simulink model "generic"  (R2022b)
settings: Solver=ode45  StartTime=0.0  StopTime=inf  RelTol=1e-3  EnableMultiTasking=on
values from neighbouring files (symbols this model uses):
  A = cell2mat(A_cell)    [MPCController1.m]    (also in MPC_Fmincon.m)
  B = cell2mat(B_cell)    [MPCController1.m]    (also in MPC_Fmincon.m)
  brake_select = ones(length(speed), length(steering_angle))    [TwoDLook_uptable.m]
  curvature = 0.000:0.001:1    [TwoDLook_uptable.m]
  m = 1600    [MPCController1.m]    (also in MPCController2.m; MPC_Fmincon.m)
  speed = 0:0.1:100    [TwoDLook_uptable.m]
undefined symbols (not defined in the file or in its folder): Amplifier, DiscIntNeverNeededParam, K_d_yawrate, K_dsteering, k_speed, k_stanley, kd, ki, kp, path_curvature
libraries: CarMaker4SL x97, simulink x6, cstblocks x6, simulink_extras x4, autolibshared x1, mpcadaslib x1
(part 2 of 6)

== system generic/CarMaker/VehicleControl/CreateBus VhclCtrl1/MPC_steering_controllers ==
  Lateral_dev : Inport
  Dev_angle : Inport  Port=2
  Amplifyer : Gain  Gain=Amplifier
  Amplifyer1 : Gain  Gain=2
  Amplifyer2 : Gain  Gain=-3
  Bus Selector1 : BusSelector  OutputSignals=Path.tx,Path.ty,Path,Path.DevAng,Path.CurveXY
  Constant1 : Constant  Value=3
  Constant2 : Constant  Value=0
  Demux : Demux  Outputs=5
  Discrete-Time Integrator : DiscreteIntegrator  SampleTime=-1  ICPrevOutput=DiscIntNeverNeededParam  ICPrevScaledInput=DiscIntNeverNeededParam
  MATLAB System : MATLABSystem  Commented=on  System=MPCController  Nx=5  Nu=1  Ny=2  Np=20  Nc=10  T=0.01  lf=1.488  lr=1.487  Ccf=66900  Ccr=62700  m=1600  g=9.81  I=2986.624  x_dot=15  Q=diag( [ 2000, 0, 0, 10000, 0 ] )  R=5 * 10 ^ 5  Row=1000  umin=-0.6  umax=0.6  delta_umin=-0.06  delta_umax=0.06  ycmax=[ 0.2; 1000 ]  ycmin=[ -0.2; -1000 ]  SimulateUsing=Code generation
      mask Type: MPCController
      mask Display:
      | disp('MPCController');
      | port_label('input',1,'y_dot');
      | port_label('input',2,'phi');
      | port_label('input',3,'phi_dot');
      | port_label('input',4,'Y');
      | port_label('input',5,'X');
      | port_label('output',1,'delta_f');
      | port_label('output',2,'state_k1');
  Multiport Switch : MultiPortSwitch  SaturateOnIntegerOverflow=off  InputSameDT=off
  Mux1 : Mux  Inputs=5
  Mux3 : Mux  Inputs=1
  Product : Product
  Radians to Degrees : simulink_extras/Transformations/Radians to Degrees
  Radians to Degrees1 : simulink_extras/Transformations/Radians to Degrees
  Read CM Dict : CarMaker4SL/Read CM Dict  xname=Sensor.Road.VehSensor_0.Path.DevAng  xsync=off  xstime=Continuous
  Read CM Dict1 : CarMaker4SL/Read CM Dict  xname=Car.Road.Path.DevDist  xsync=off  xstime=Continuous
  Read CM Dict8 : CarMaker4SL/Read CM Dict  xname=Vhcl.v  xsync=off  xstime=Continuous
  Road Sensor1 : CarMaker4SL/Sensors/Road Sensor  xname=0  xstime=Continuous
      settings: SourceProductName=CarMaker4SL
  S-Function1 : S-Function  Commented=on  FunctionName=MPC_Fmincon  SFunctionDeploymentMode=off  EnableBusSupport=off
  State_space_system_variables : Subsystem
  Subsystem : Subsystem  Commented=on
  Terminator : Terminator
  Terminator1 : Terminator  Commented=on
  Terminator2 : Terminator
  Terminator3 : Terminator
  Tradition_MPC : Subsystem
  steering : Outport
  wires:
  Constant2/1 -> Road Sensor1/1
  Demux/1 -> MATLAB System/4
  Bus Selector1/5 -> Product/2  "<CurveXY>"
  Bus Selector1/3 -> Terminator1/1  "<Path>"
  Road Sensor1/1 -> Terminator/1
  Road Sensor1/2 -> Bus Selector1/1
  Mux3/1 -> S-Function1/1, Demux/1
  Read CM Dict8/1 -> Product/1
  Bus Selector1/1 -> Mux1/5  "<tx>"
  Bus Selector1/2 -> State_space_system_variables/2(<ty>), Mux1/4  "<ty>"
  Product/1 -> Discrete-Time Integrator/1, Radians to Degrees1/1
  Discrete-Time Integrator/1 -> Radians to Degrees/1
  Radians to Degrees/1 -> State_space_system_variables/1(Yaw_ref_deg), Mux1/2
  Constant1/1 -> Multiport Switch/1
  Radians to Degrees1/1 -> Mux1/3
  State_space_system_variables/1(x) -> Mux3/1
  Demux/5 -> MATLAB System/3
  Demux/3 -> MATLAB System/1
  State_space_system_variables/2(Lateral_velocity) -> Mux1/1
  Read CM Dict/1 -> Amplifyer/1
  Mux1/1 -> Terminator2/1  "u"
  Read CM Dict1/1 -> ?
  Amplifyer/1 -> ?  "Dev_angle"
  Demux/2 -> MATLAB System/5
  Demux/4 -> MATLAB System/2
  Amplifyer1/1 -> Tradition_MPC/1(Lateral_deviation)  "Dev_angle"
  Amplifyer2/1 -> Tradition_MPC/2(Dev_angle)  "Dev_angle"
  MATLAB System/1 -> Multiport Switch/3
  Multiport Switch/1 -> steering/1
  MATLAB System/2 -> Terminator3/1
  S-Function1/1 -> Multiport Switch/2
  Tradition_MPC/1(steering_cmd) -> Multiport Switch/4
  Lateral_dev/1 -> Amplifyer1/1
  Dev_angle/1 -> Amplifyer2/1

== system generic/CarMaker/VehicleControl/CreateBus VhclCtrl1/PID steering controller ==
  Lateral_error : Inport
  Add : Sum  Inputs=+++
  Dervative : Subsystem
  Discrete-Time Integrator : DiscreteIntegrator  SampleTime=-1  ICPrevOutput=DiscIntNeverNeededParam  ICPrevScaledInput=DiscIntNeverNeededParam
  Gain : Gain  Gain=1.1
  Gain1 : Gain  Gain=0.9
  steering_cmd : Outport
  wires:
  Lateral_error/1 -> Gain1/1, Gain/1, Dervative/1(Error)
  Discrete-Time Integrator/1 -> Add/1
  Gain1/1 -> Discrete-Time Integrator/1
  Gain/1 -> Add/2
  Add/1 -> steering_cmd/1
  Dervative/1(Dervative term) -> Add/3

== system generic/CarMaker/VehicleControl/CreateBus VhclCtrl1/Smoothing ==
  Signal_In : Inport
  Add : Sum  Inputs=++++
  Delay : Delay  InitialCondition=0.1
  Delay1 : Delay  DelayLength=4  InitialCondition=0.1
  Delay2 : Delay  DelayLength=5  InitialCondition=0.1
  Gain : Gain  Gain=0.35
  Gain1 : Gain  Gain=0.25
  Gain2 : Gain  Gain=0.25
  Gain3 : Gain  Gain=0.15
  Signal_Out : Outport  VectorParamsAs1DForOutWhenUnconnected=off
  wires:
  Gain1/1 -> Add/2
  Signal_In/1 -> Gain/1
  Delay/1 -> Gain1/1
  Gain/1 -> Add/1
  Delay1/1 -> Gain2/1
  Add/1 -> Delay2/1, Delay1/1, Delay/1, Signal_Out/1
  Gain2/1 -> Add/3
  Delay2/1 -> Gain3/1
  Gain3/1 -> Add/4

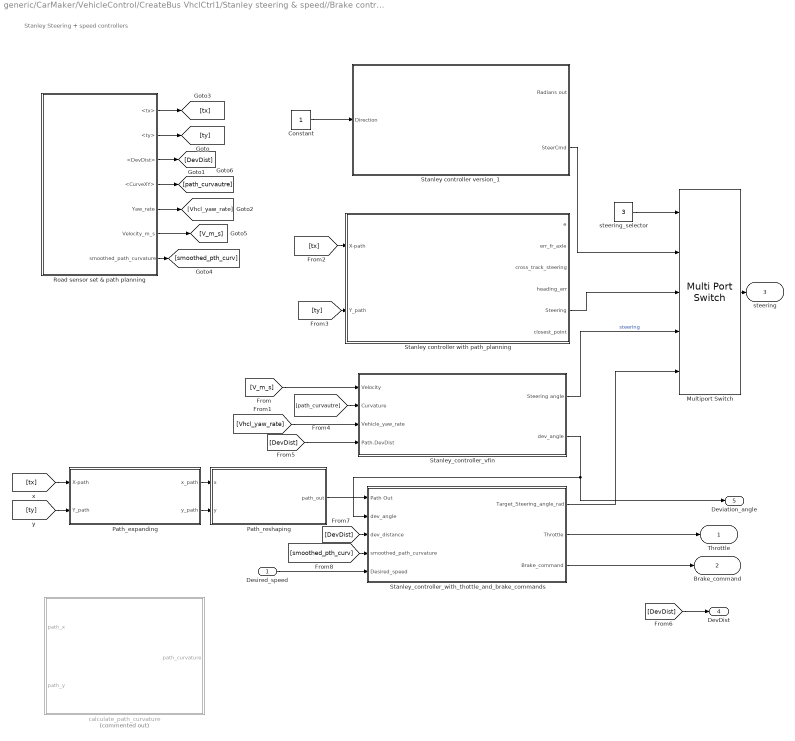
== system generic/CarMaker/VehicleControl/CreateBus VhclCtrl1/Stanley steering & speed//Brake controller ==
  note: Stanley Steering + speed controllers
  Desired_speed : Inport
  " Path_expanding" : Subsystem
  Constant : Constant
  Multiport Switch : MultiPortSwitch  Inputs=4  SaturateOnIntegerOverflow=off  InputSameDT=off
  Path_reshaping : MATLAB Function  TreatAsAtomicUnit=on
  Road sensor set & path planning : Subsystem  Variant=on  VariantControlMode=label  VariantControl=Choice  LabelModeActiveChoice=Choice
  Stanley controller version_1 : Subsystem  Variant=on  VariantControlMode=label  VariantControl=Choice  LabelModeActiveChoice=Choice
  Stanley controller with path_planning : Subsystem  Variant=on  VariantControlMode=label  VariantControl=Choice  LabelModeActiveChoice=Choice
  Stanley_controller_vfin : Subsystem  Variant=on  VariantControlMode=label  VariantControl=Choice  LabelModeActiveChoice=Choice
  Stanley_controller_with_thottle_and_brake_commands : Subsystem
  calculate_path_curvature : Subsystem  Commented=on  Variant=on  VariantControlMode=label  VariantControl=Choice  LabelModeActiveChoice=Choice
  steering_selector : Constant  Value=3
  Throttle : Outport
  Brake_command : Outport  Port=2
  steering : Outport  Port=3
  DevDist : Outport  Port=4
  Deviation_angle : Outport  Port=5
  wires:
  [tx] -> " Path_expanding"/1(X-path)
  [ty] -> " Path_expanding"/2(Y_path)
  [tx] -> Stanley controller with path_planning/1(X-path)
  [ty] -> Stanley controller with path_planning/2(Y_path)
  Road sensor set & path planning/1(<tx>) -> [tx]
  Road sensor set & path planning/2(<ty>) -> [ty]
  Road sensor set & path planning/3(<DevDist>) -> [DevDist]
  Road sensor set & path planning/4(<CurveXY>) -> [path_curvautre]
  Road sensor set & path planning/5(Yaw_rate) -> [Vhcl_yaw_rate]
  [path_curvautre] -> Stanley_controller_vfin/2(Curvature)
  Stanley_controller_vfin/1(Steering angle) -> Multiport Switch/4  "steering"
  Constant/1 -> Stanley controller version_1/1(Direction)
  steering_selector/1 -> Multiport Switch/1
  Stanley controller version_1/2(SteerCmd) -> Multiport Switch/2
  Stanley controller with path_planning/5(Steering) -> Multiport Switch/3
  Path_reshaping/1(path_out) -> Stanley_controller_with_thottle_and_brake_commands/1(Path Out)
  Stanley_controller_vfin/2(dev_angle) -> Deviation_angle/1, Stanley_controller_with_thottle_and_brake_commands/2(dev_angle)
  " Path_expanding"/1(x_path) -> Path_reshaping/1(x)
  " Path_expanding"/2(y_path) -> Path_reshaping/2(y)
  Stanley_controller_with_thottle_and_brake_commands/2(Throttle) -> Throttle/1
  Stanley_controller_with_thottle_and_brake_commands/3(Brake_command) -> Brake_command/1
  Stanley_controller_with_thottle_and_brake_commands/1(Target_Steering_angle_rad) -> Multiport Switch/5
  [V_m_s] -> Stanley_controller_vfin/1(Velocity)
  [Vhcl_yaw_rate] -> Stanley_controller_vfin/3(Vehicle_yaw_rate)
  [DevDist] -> Stanley_controller_vfin/4(Path.DevDist)
  Road sensor set & path planning/6(Velocity_m_s) -> [V_m_s]
  [DevDist] -> DevDist/1
  Multiport Switch/1 -> steering/1
  [DevDist] -> Stanley_controller_with_thottle_and_brake_commands/3(dev_distance)
  Road sensor set & path planning/7(smoothed_path_curvature) -> [smoothed_pth_curv]
  [smoothed_pth_curv] -> Stanley_controller_with_thottle_and_brake_commands/4(smoothed_path_curvature)
  Desired_speed/1 -> Stanley_controller_with_thottle_and_brake_commands/5(Desired_speed)

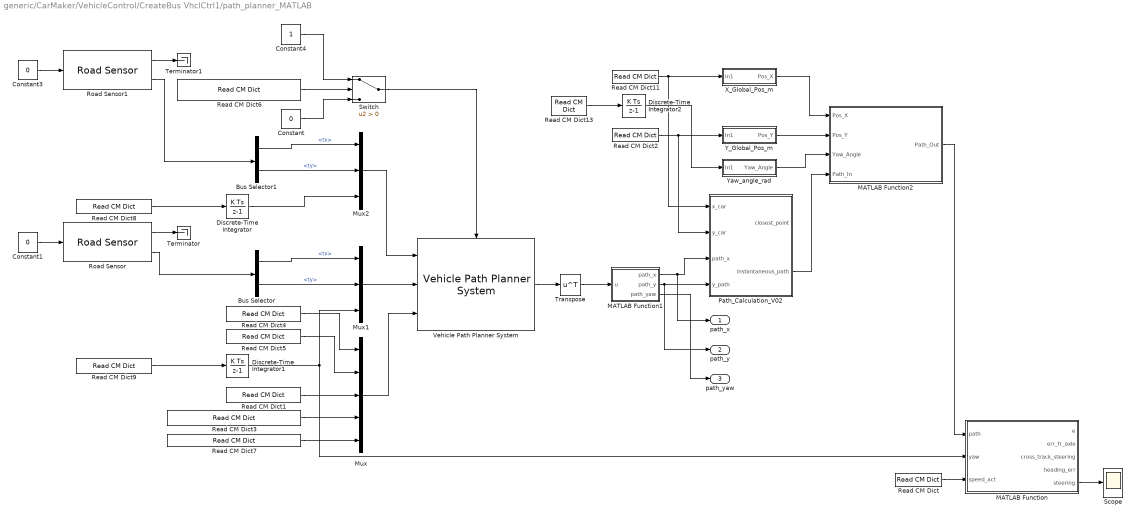
== system generic/CarMaker/VehicleControl/CreateBus VhclCtrl1/path_planner_MATLAB ==
  Bus Selector : BusSelector  OutputSignals=Path.tx,Path.ty
  Bus Selector1 : BusSelector  OutputSignals=Path.tx,Path.ty
  Constant : Constant  Value=0
  Constant1 : Constant  Value=0
  Constant3 : Constant  Value=0
  Constant4 : Constant
  Discrete-Time Integrator : DiscreteIntegrator  SampleTime=-1  ICPrevOutput=DiscIntNeverNeededParam  ICPrevScaledInput=DiscIntNeverNeededParam
  Discrete-Time Integrator1 : DiscreteIntegrator  SampleTime=-1  ICPrevOutput=DiscIntNeverNeededParam  ICPrevScaledInput=DiscIntNeverNeededParam
  Discrete-Time Integrator2 : DiscreteIntegrator  SampleTime=-1  ICPrevOutput=DiscIntNeverNeededParam  ICPrevScaledInput=DiscIntNeverNeededParam
  MATLAB Function : MATLAB Function  TreatAsAtomicUnit=on
  MATLAB Function1 : MATLAB Function  TreatAsAtomicUnit=on
  MATLAB Function2 : MATLAB Function  TreatAsAtomicUnit=on
  Mux : Mux  Inputs=5
  Mux1 : Mux  Inputs=3
  Mux2 : Mux  Inputs=3
  Path_Calculation_V02 : MATLAB Function  TreatAsAtomicUnit=on
  Read CM Dict : CarMaker4SL/Read CM Dict  xname=Vhcl.v  xsync=off  xstime=Continuous
  Read CM Dict1 : CarMaker4SL/Read CM Dict  xname=Traffic.T00.rz  xsync=off  xstime=Continuous
  Read CM Dict11 : CarMaker4SL/Read CM Dict  xname=Car.Gen.tx  xsync=off  xstime=Continuous
  Read CM Dict13 : CarMaker4SL/Read CM Dict  xname=Car.YawRate  xsync=off  xstime=Continuous
  Read CM Dict2 : CarMaker4SL/Read CM Dict  xname=Car.Gen.ty  xsync=off  xstime=Continuous
  Read CM Dict3 : CarMaker4SL/Read CM Dict  xname=Sensor.Radar.VehSensor_6.Obj0.Length  xsync=off  xstime=Continuous
  Read CM Dict4 : CarMaker4SL/Read CM Dict  xname=Traffic.T00.tx  xsync=off  xstime=Continuous
  Read CM Dict5 : CarMaker4SL/Read CM Dict  xname=Traffic.T00.ty  xsync=off  xstime=Continuous
  Read CM Dict6 : CarMaker4SL/Read CM Dict  xname=Sensor.Radar.VehSensor_6.Obj0.ProbObst  xsync=off  xstime=Continuous
  Read CM Dict7 : CarMaker4SL/Read CM Dict  xname=Sensor.Radar.VehSensor_6.Obj0.Width  xsync=off  xstime=Continuous
  Read CM Dict8 : CarMaker4SL/Read CM Dict  xname=Car.YawRate  xsync=off  xstime=Continuous
  Read CM Dict9 : CarMaker4SL/Read CM Dict  xname=Car.YawRate  xsync=off  xstime=Continuous
  Road Sensor : CarMaker4SL/Sensors/Road Sensor  xname=0  xstime=Continuous
      settings: SourceProductName=CarMaker4SL
  Road Sensor1 : CarMaker4SL/Sensors/Road Sensor  xname=0  xstime=Continuous
      settings: SourceProductName=CarMaker4SL
  Scope : Scope
  Switch : Switch  Criteria=u2 > Threshold  SaturateOnIntegerOverflow=off  InputSameDT=off
  Terminator : Terminator
  Terminator1 : Terminator
  Transpose : Math  Operator=transpose
  Vehicle Path Planner System : mpcadaslib/Vehicle Path Planner System  egoLength=4.7  egoWidth=1.8  wheelbase=2.8  dist2Center=1.4  numObs=1  obsMat=zeros(1,5)  obs_ext=on  minDist=1  Ts=1  pPlanning=20  v_range=[-20,30]  v_ext=off  steer_range=[-pi/4,pi/4]  steer_ext=off  suboptimal=off  maxiter=200  output_exitflag=off
      settings: LibrarySourceBlock=mpclib/Automated Driving/Vehicle Path Planner System
  X_Global_Pos_m : Subsystem
  Y_Global_Pos_m : Subsystem
  Yaw_angle_rad : Subsystem
  path_x : Outport
  path_y : Outport  Port=2
  path_yaw : Outport  Port=3
  wires:
  Constant3/1 -> Road Sensor1/1
  Mux1/1 -> Vehicle Path Planner System/2
  Road Sensor/1 -> Terminator/1
  Road Sensor1/1 -> Terminator1/1
  Constant1/1 -> Road Sensor/1
  Bus Selector1/2 -> Mux2/2  "<ty>"
  Read CM Dict9/1 -> Discrete-Time Integrator1/1
  Road Sensor/2 -> Bus Selector/1
  Road Sensor1/2 -> Bus Selector1/1
  Read CM Dict8/1 -> Discrete-Time Integrator/1
  MATLAB Function2/1(Path_Out) -> MATLAB Function/1(path)
  Constant4/1 -> Switch/1
  Read CM Dict6/1 -> Switch/2
  Constant/1 -> Switch/3
  MATLAB Function1/1(path_x) -> Path_Calculation_V02/3(path_x), path_x/1
  Bus Selector1/1 -> Mux2/1  "<tx>"
  Discrete-Time Integrator/1 -> Mux2/3
  Bus Selector/1 -> Mux1/1  "<tx>"
  Bus Selector/2 -> Mux1/2  "<ty>"
  X_Global_Pos_m/1(Pos_X) -> MATLAB Function2/1(Pos_X)
  Read CM Dict4/1 -> Mux/1
  Read CM Dict5/1 -> Mux/2
  Read CM Dict11/1 -> Path_Calculation_V02/1(x_car), X_Global_Pos_m/1(In1)
  Discrete-Time Integrator1/1 -> MATLAB Function/2(yaw), Mux1/3
  Read CM Dict1/1 -> Mux/3
  Read CM Dict3/1 -> Mux/4
  Y_Global_Pos_m/1(Pos_Y) -> MATLAB Function2/2(Pos_Y)
  Read CM Dict7/1 -> Mux/5
  Transpose/1 -> MATLAB Function1/1(u)
  Switch/1 -> Vehicle Path Planner System/Enable
  Mux2/1 -> Vehicle Path Planner System/1
  Mux/1 -> Vehicle Path Planner System/3
  Vehicle Path Planner System/1 -> Transpose/1
  Read CM Dict13/1 -> Discrete-Time Integrator2/1
  Discrete-Time Integrator2/1 -> Yaw_angle_rad/1(In1)
  Read CM Dict2/1 -> Path_Calculation_V02/2(y_car), Y_Global_Pos_m/1(In1)
  MATLAB Function/5(steering) -> Scope/1
  MATLAB Function1/2(path_y) -> path_y/1, Path_Calculation_V02/4(y_path)
  MATLAB Function1/3(path_yaw) -> path_yaw/1
  Yaw_angle_rad/1(Yaw_Angle) -> MATLAB Function2/3(Yaw_Angle)
  Path_Calculation_V02/2(instantaneous_path) -> MATLAB Function2/4(Path_In)
  Read CM Dict/1 -> MATLAB Function/3(speed_act)

== system generic/CarMaker/IPG Vehicle/CarAndTrailer/CarAndTrailerUpd/CreateBus Brake.IF.In ==
  In : Inport
  BusCreator : BusCreator  Inputs=9
  Demux : Demux  Outputs=9
      settings: DisplayOption=none
  Out : Outport  VectorParamsAs1DForOutWhenUnconnected=off
  wires:
  Demux/9 -> BusCreator/9  "Brake IF Trq_Reg RR"
  Demux/8 -> BusCreator/8  "Brake IF Trq_Reg RL"
  Demux/7 -> BusCreator/7  "Brake IF Trq_Reg FR"
  Demux/6 -> BusCreator/6  "Brake IF Trq_Reg FL"
  Demux/5 -> BusCreator/5  "Brake IF Trq_Reg_max RR"
  Demux/4 -> BusCreator/4  "Brake IF Trq_Reg_max RL"
  Demux/3 -> BusCreator/3  "Brake IF Trq_Reg_max FR"
  Demux/2 -> BusCreator/2  "Brake IF Trq_Reg_max FL"
  Demux/1 -> BusCreator/1  "Brake IF T_env"
  BusCreator/1 -> Out/1
  In/1 -> Demux/1

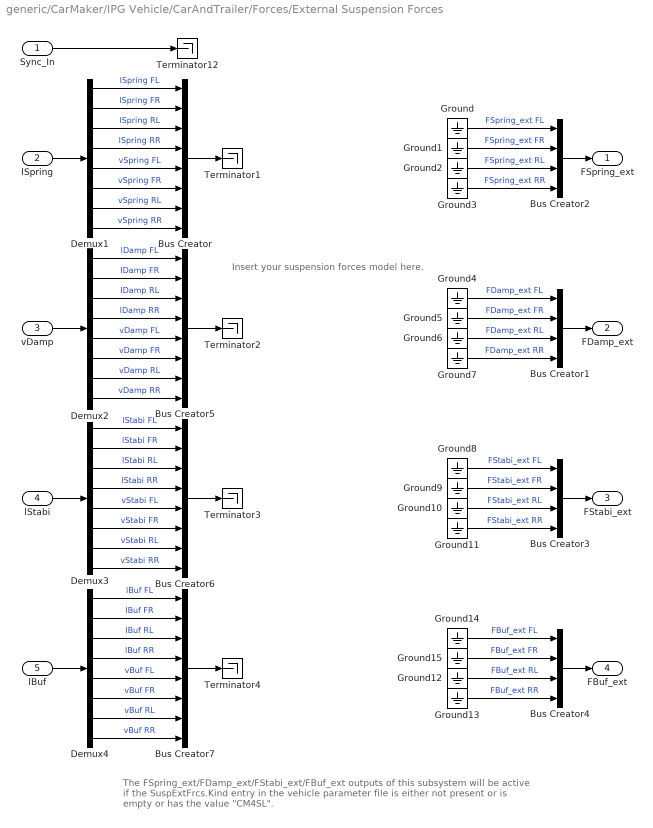
== system generic/CarMaker/IPG Vehicle/CarAndTrailer/Forces/External Suspension Forces ==
  note: The FSpring_ext/FDamp_ext/FStabi_ext/FBuf_ext outputs of this subsystem will be
      | active if the SuspExtFrcs.Kind entry in the vehicle parameter file
      | is either not present or is empty or has the value "CM4SL".
  note: Insert your suspension forces model here.
  Sync_In : Inport
  lSpring : Inport  Port=2
  vDamp : Inport  Port=3
  lStabi : Inport  Port=4
  lBuf : Inport  Port=5
  Bus Creator{,5..7} (4 alike) : BusCreator  Inputs=8
  Bus Creator{1..4} (4 alike) : BusCreator  Inputs=4
  Demux{1..4} (4 alike) : Demux  Outputs=8
      settings: DisplayOption=none
  Ground{,1..15} (16 alike) : Ground
  Terminator{1..4,12} (5 alike) : Terminator
  FSpring_ext : Outport  VectorParamsAs1DForOutWhenUnconnected=off
  FDamp_ext : Outport  Port=2  VectorParamsAs1DForOutWhenUnconnected=off
  FStabi_ext : Outport  Port=3  VectorParamsAs1DForOutWhenUnconnected=off
  FBuf_ext : Outport  Port=4  VectorParamsAs1DForOutWhenUnconnected=off
  wires:
  Bus Creator7/1 -> Terminator4/1
  Bus Creator6/1 -> Terminator3/1
  Bus Creator5/1 -> Terminator2/1
  Bus Creator/1 -> Terminator1/1
  Demux4/8 -> Bus Creator7/8  "vBuf RR"
  Demux4/7 -> Bus Creator7/7  "vBuf RL"
  Demux4/6 -> Bus Creator7/6  "vBuf FR"
  Demux4/5 -> Bus Creator7/5  "vBuf FL"
  Demux3/8 -> Bus Creator6/8  "vStabi RR"
  Demux3/7 -> Bus Creator6/7  "vStabi RL"
  Demux3/6 -> Bus Creator6/6  "vStabi FR"
  Demux3/5 -> Bus Creator6/5  "vStabi FL"
  Demux2/8 -> Bus Creator5/8  "vDamp RR"
  Demux2/7 -> Bus Creator5/7  "vDamp RL"
  Demux2/6 -> Bus Creator5/6  "vDamp FR"
  Demux2/5 -> Bus Creator5/5  "vDamp FL"
  Demux1/8 -> Bus Creator/8  "vSpring RR"
  Demux1/7 -> Bus Creator/7  "vSpring RL"
  Demux1/6 -> Bus Creator/6  "vSpring FR"
  Demux1/5 -> Bus Creator/5  "vSpring FL"
  Demux2/4 -> Bus Creator5/4  "lDamp RR"
  Demux2/3 -> Bus Creator5/3  "lDamp RL"
  Demux2/2 -> Bus Creator5/2  "lDamp FR"
  Demux2/1 -> Bus Creator5/1  "lDamp FL"
  Demux1/4 -> Bus Creator/4  "lSpring RR"
  Demux1/3 -> Bus Creator/3  "lSpring RL"
  Demux1/2 -> Bus Creator/2  "lSpring FR"
  Demux1/1 -> Bus Creator/1  "lSpring FL"
  Demux3/4 -> Bus Creator6/4  "lStabi RR"
  Demux3/3 -> Bus Creator6/3  "lStabi RL"
  Demux3/2 -> Bus Creator6/2  "lStabi FR"
  Demux3/1 -> Bus Creator6/1  "lStabi FL"
  lStabi/1 -> Demux3/1
  vDamp/1 -> Demux2/1
  lSpring/1 -> Demux1/1
  Demux4/4 -> Bus Creator7/4  "lBuf RR"
  Demux4/3 -> Bus Creator7/3  "lBuf RL"
  Demux4/2 -> Bus Creator7/2  "lBuf FR"
  Demux4/1 -> Bus Creator7/1  "lBuf FL"
  lBuf/1 -> Demux4/1
  Ground14/1 -> Bus Creator4/1  "FBuf_ext FL"
  Ground15/1 -> Bus Creator4/2  "FBuf_ext FR"
  Ground12/1 -> Bus Creator4/3  "FBuf_ext RL"
  Ground13/1 -> Bus Creator4/4  "FBuf_ext RR"
  Bus Creator4/1 -> FBuf_ext/1
  Sync_In/1 -> Terminator12/1
  Bus Creator2/1 -> FSpring_ext/1
  Ground/1 -> Bus Creator2/1  "FSpring_ext FL"
  Ground1/1 -> Bus Creator2/2  "FSpring_ext FR"
  Ground2/1 -> Bus Creator2/3  "FSpring_ext RL"
  Ground3/1 -> Bus Creator2/4  "FSpring_ext RR"
  Ground4/1 -> Bus Creator1/1  "FDamp_ext FL"
  Ground5/1 -> Bus Creator1/2  "FDamp_ext FR"
  Ground6/1 -> Bus Creator1/3  "FDamp_ext RL"
  Ground7/1 -> Bus Creator1/4  "FDamp_ext RR"
  Bus Creator1/1 -> FDamp_ext/1
  Ground8/1 -> Bus Creator3/1  "FStabi_ext FL"
  Ground9/1 -> Bus Creator3/2  "FStabi_ext FR"
  Ground10/1 -> Bus Creator3/3  "FStabi_ext RL"
  Ground11/1 -> Bus Creator3/4  "FStabi_ext RR"
  Bus Creator3/1 -> FStabi_ext/1

== system generic/CarMaker/IPG Vehicle/CarAndTrailer/Forces/Suspension Forces ==
  note: <Your model here>
  note: <Your model here>
  Sync_In : Inport
  lSpring : Inport  Port=2
  vDamp : Inport  Port=3
  lStabi : Inport  Port=4
  lBuf : Inport  Port=5
  Bus Creator{,1..3,8..10} (7 alike) : BusCreator  Inputs=4
  Bus Creator{4..7} (4 alike) : BusCreator  Inputs=6
  Demux{,1..5} (6 alike) : Demux
  Demux{6..9} (4 alike) : Demux  Outputs=6
  Suspension Control Unit : S-Function  FunctionName=CM_Sfun  Parameters='ForcesSuspControl'  SFunctionDeploymentMode=off  EnableBusSupport=off
  Suspension Force Elements : S-Function  FunctionName=CM_Sfun  Parameters='ForcesSusp'  SFunctionDeploymentMode=off  EnableBusSupport=off
  Suspension Force Elements Update : S-Function  FunctionName=CM_Sfun  Parameters='ForcesSuspUpd'  SFunctionDeploymentMode=off  EnableBusSupport=off
  Sync_Out : Outport  VectorParamsAs1DForOutWhenUnconnected=off
  wires:
  vDamp/1 -> Bus Creator8/2
  lStabi/1 -> Bus Creator8/3
  lBuf/1 -> Bus Creator8/4
  lSpring/1 -> Bus Creator8/1
  Bus Creator8/1 -> Suspension Control Unit/2, Suspension Force Elements/2
  Sync_In/1 -> Suspension Control Unit/1
  Suspension Control Unit/1 -> Suspension Force Elements/1
  Suspension Force Elements/1 -> Suspension Force Elements Update/1
  Suspension Force Elements Update/1 -> Sync_Out/1
  Bus Creator4/1 -> Bus Creator10/1
  Bus Creator5/1 -> Bus Creator10/2
  Bus Creator6/1 -> Bus Creator10/3
  Bus Creator7/1 -> Bus Creator10/4
  Demux6/1 -> Bus Creator4/1  "FL SpringForce"
  Demux9/1 -> Bus Creator7/1  "RR SpringForce"
  Demux9/2 -> Bus Creator7/2  "RR DamperForce"
  Demux9/3 -> Bus Creator7/3  "RR StabiForce"
  Demux9/4 -> Bus Creator7/4  "RR BufferForce"
  Demux9/5 -> Bus Creator7/5  "RR ParasiticStiffForce"
  Demux9/6 -> Bus Creator7/6  "RR ParasiticFricForce"
  Demux8/1 -> Bus Creator6/1  "RL SpringForce"
  Demux8/2 -> Bus Creator6/2  "RL DamperForce"
  Demux8/4 -> Bus Creator6/4  "RL BufferForce"
  Demux8/5 -> Bus Creator6/5  "RL ParasiticStiffForce"
  Demux8/6 -> Bus Creator6/6  "RL ParasiticFricForce"
  Demux8/3 -> Bus Creator6/3  "RL StabiForce"
  Demux7/1 -> Bus Creator5/1  "FR SpringForce"
  Demux7/2 -> Bus Creator5/2  "FR DamperForce"
  Demux7/3 -> Bus Creator5/3  "FR StabiForce"
  Demux7/4 -> Bus Creator5/4  "FR BufferForce"
  Demux7/5 -> Bus Creator5/5  "FR ParasiticStiffForce"
  Demux7/6 -> Bus Creator5/6  "FR ParasiticFricForce"
  Demux6/2 -> Bus Creator4/2  "FL DamperForce"
  Demux6/3 -> Bus Creator4/3  "FL StabiForce"
  Demux6/4 -> Bus Creator4/4  "FL BufferForce"
  Demux6/5 -> Bus Creator4/5  "FL ParasiticStiffForce"
  Demux6/6 -> Bus Creator4/6  "FL ParasiticFricForce"
  Bus Creator10/1 -> Suspension Force Elements Update/2
  Demux/1 -> Demux2/1  "FL"
  Bus Creator1/1 -> Bus Creator9/2
  Demux/2 -> Demux3/1  "FR"
  Bus Creator2/1 -> Bus Creator9/3
  Demux/3 -> Demux4/1  "RL"
  Bus Creator3/1 -> Bus Creator9/4
  Demux2/1 -> Bus Creator/1  "FL SpringCtrlOut"
  Demux/4 -> Demux5/1  "RR"
  Demux5/1 -> Bus Creator3/1  "RR SpringCtrlOut"
  Demux5/2 -> Bus Creator3/2  "RR DamperCtrlOut"
  Demux5/3 -> Bus Creator3/3  "RR StabiCtrlOut"
  Demux5/4 -> Bus Creator3/4  "RR BufferCtrlOut"
  Demux4/1 -> Bus Creator2/1  "RL SpringCtrlOut"
  Demux4/2 -> Bus Creator2/2  "RL DamperCtrlOut"
  Demux4/4 -> Bus Creator2/4  "RL BufferCtrlOut"
  Demux4/3 -> Bus Creator2/3  "RL StabiCtrlOut"
  Demux3/1 -> Bus Creator1/1  "FR SpringCtrlOut"
  Demux3/2 -> Bus Creator1/2  "FR DamperCtrlOut"
  Demux3/3 -> Bus Creator1/3  "FR StabiCtrlOut"
  Demux3/4 -> Bus Creator1/4  "FR BufferCtrlOut"
  Demux2/2 -> Bus Creator/2  "FL DamperCtrlOut"
  Demux2/3 -> Bus Creator/3  "FL StabiCtrlOut"
  Demux2/4 -> Bus Creator/4  "FL BufferCtrlOut"
  Suspension Control Unit/2 -> Demux/1
  Bus Creator9/1 -> Suspension Force Elements/3
  Bus Creator/1 -> Bus Creator9/1
  Suspension Force Elements/2 -> Demux1/1
  Demux1/1 -> Demux6/1  "FL"
  Demux1/2 -> Demux7/1  "FR"
  Demux1/3 -> Demux8/1  "RL"
  Demux1/4 -> Demux9/1  "RR"

== system generic/CarMaker/IPG Vehicle/CarAndTrailer/Forces/Tires ==
  note: The TireXX_Out signals will only be used if FileIdent is "CarMaker-Tire-CM4SL" in the tire parameter file!
      | An example parameter file can be found in Data/Tire/DT_CM4SL_UserTire.
  Sync_In : Inport
  TireFL_In : Inport  Port=2
  TireFR_In : Inport  Port=3
  TireRL_In : Inport  Port=4
  TireRR_In : Inport  Port=5
  Bus Creator{1..4} (4 alike) : BusCreator  Inputs=11
  Demux{1..3,8} (4 alike) : Demux  Outputs=7
      settings: DisplayOption=none
  TireFL : Subsystem
  TireFR : Subsystem
  TireRL : Subsystem
  TireRR : Subsystem
  TireFL_Out : Outport  VectorParamsAs1DForOutWhenUnconnected=off
  TireFR_Out : Outport  Port=2  VectorParamsAs1DForOutWhenUnconnected=off
  TireRL_Out : Outport  Port=3  VectorParamsAs1DForOutWhenUnconnected=off
  TireRR_Out : Outport  Port=4  VectorParamsAs1DForOutWhenUnconnected=off
  wires:
  Sync_In/1 -> TireRR/1(Sync_In), TireRL/1(Sync_In), TireFR/1(Sync_In), TireFL/1(Sync_In)
  Bus Creator4/1 -> TireRR_Out/1
  Bus Creator2/1 -> TireRL_Out/1
  Bus Creator1/1 -> TireFR_Out/1
  Demux3/5 -> TireRR/6(Rim_turnv)  "Tire_In Rim_turnv"
  Demux3/4 -> TireRR/5(Rim_rotv)  "Tire_In Rim_rotv"
  Demux3/1 -> TireRR/2(Load)  "Tire_In Load"
  Demux3/7 -> TireRR/8(muRoad)  "Tire_In mu"
  Demux3/6 -> TireRR/7(InclinAngle)  "Tire_In Camber"
  Demux3/2 -> TireRR/3(vxtrans)  "Tire_In vxtrans"
  Demux3/3 -> TireRR/4(vytrans)  "Tire_In vytrans"
  TireRR/11(AlignTrq) -> Bus Creator4/11  "Tire_Out AlignTrq"
  TireRR/10(RollResist) -> Bus Creator4/10  "Tire_Out RollResist"
  TireRR/9(OverturnTrq) -> Bus Creator4/9  "Tire_Out OverturnTrq"
  TireRR/8(LoadFrc) -> Bus Creator4/8  "Tire_Out LoadFrc"
  TireRR/7(SideFrc) -> Bus Creator4/7  "Tire_Out SideFrc"
  TireRR/6(LongFrc) -> Bus Creator4/6  "Tire_Out LongFrc"
  TireRR/5(vBelt) -> Bus Creator4/5  "Tire_Out vBelt"
  TireRR/4(rBelt_eff) -> Bus Creator4/4  "Tire_Out rBelt_eff"
  TireRR/3(TurnSlp) -> Bus Creator4/3  "Tire_Out TurnSlp"
  TireRR/1(Slp) -> Bus Creator4/1  "Tire_Out Slp"
  TireRR/2(Alpha) -> Bus Creator4/2  "Tire_Out Alpha"
  Demux2/5 -> TireRL/6(Rim_turnv)  "Tire_In Rim_turnv"
  Demux2/4 -> TireRL/5(Rim_rotv)  "Tire_In Rim_rotv"
  Demux2/1 -> TireRL/2(Load)  "Tire_In Load"
  Demux2/7 -> TireRL/8(muRoad)  "Tire_In mu"
  Demux2/6 -> TireRL/7(InclinAngle)  "Tire_In Camber"
  Demux2/2 -> TireRL/3(vxtrans)  "Tire_In vxtrans"
  Demux2/3 -> TireRL/4(vytrans)  "Tire_In vytrans"
  TireRL/11(AlignTrq) -> Bus Creator2/11  "Tire_Out AlignTrq"
  TireRL/10(RollResist) -> Bus Creator2/10  "Tire_Out RollResist"
  TireRL/9(OverturnTrq) -> Bus Creator2/9  "Tire_Out OverturnTrq"
  TireRL/8(LoadFrc) -> Bus Creator2/8  "Tire_Out LoadFrc"
  TireRL/7(SideFrc) -> Bus Creator2/7  "Tire_Out SideFrc"
  TireRL/6(LongFrc) -> Bus Creator2/6  "Tire_Out LongFrc"
  TireRL/5(vBelt) -> Bus Creator2/5  "Tire_Out vBelt"
  TireRL/4(rBelt_eff) -> Bus Creator2/4  "Tire_Out rBelt_eff"
  TireRL/3(TurnSlp) -> Bus Creator2/3  "Tire_Out TurnSlp"
  TireRL/1(Slp) -> Bus Creator2/1  "Tire_Out Slp"
  TireRL/2(Alpha) -> Bus Creator2/2  "Tire_Out Alpha"
  Demux1/5 -> TireFR/6(Rim_turnv)  "Tire_In Rim_turnv"
  Demux1/4 -> TireFR/5(Rim_rotv)  "Tire_In Rim_rotv"
  Demux1/1 -> TireFR/2(Load)  "Tire_In Load"
  Demux1/7 -> TireFR/8(muRoad)  "Tire_In mu"
  Demux1/6 -> TireFR/7(InclinAngle)  "Tire_In Camber"
  Demux1/2 -> TireFR/3(vxtrans)  "Tire_In vxtrans"
  Demux1/3 -> TireFR/4(vytrans)  "Tire_In vytrans"
  TireFR/11(AlignTrq) -> Bus Creator1/11  "Tire_Out AlignTrq"
  TireFR/10(RollResist) -> Bus Creator1/10  "Tire_Out RollResist"
  TireFR/9(OverturnTrq) -> Bus Creator1/9  "Tire_Out OverturnTrq"
  TireFR/8(LoadFrc) -> Bus Creator1/8  "Tire_Out LoadFrc"
  TireFR/7(SideFrc) -> Bus Creator1/7  "Tire_Out SideFrc"
  TireFR/6(LongFrc) -> Bus Creator1/6  "Tire_Out LongFrc"
  TireFR/5(vBelt) -> Bus Creator1/5  "Tire_Out vBelt"
  TireFR/4(rBelt_eff) -> Bus Creator1/4  "Tire_Out rBelt_eff"
  TireFR/3(TurnSlp) -> Bus Creator1/3  "Tire_Out TurnSlp"
  TireFR/1(Slp) -> Bus Creator1/1  "Tire_Out Slp"
  TireFR/2(Alpha) -> Bus Creator1/2  "Tire_Out Alpha"
  Demux8/5 -> TireFL/6(Rim_turnv)  "Tire_In Rim_turnv"
  Demux8/4 -> TireFL/5(Rim_rotv)  "Tire_In Rim_rotv"
  TireFL_In/1 -> Demux8/1
  Demux8/1 -> TireFL/2(Load)  "Tire_In Load"
  Demux8/7 -> TireFL/8(muRoad)  "Tire_In mu"
  Demux8/6 -> TireFL/7(InclinAngle)  "Tire_In Camber"
  Demux8/2 -> TireFL/3(vxtrans)  "Tire_In vxtrans"
  Demux8/3 -> TireFL/4(vytrans)  "Tire_In vytrans"
  TireFL/11(AlignTrq) -> Bus Creator3/11  "Tire_Out AlignTrq"
  TireFL/10(RollResist) -> Bus Creator3/10  "Tire_Out RollResist"
  TireFL/9(OverturnTrq) -> Bus Creator3/9  "Tire_Out OverturnTrq"
  TireFL/8(LoadFrc) -> Bus Creator3/8  "Tire_Out LoadFrc"
  TireFL/7(SideFrc) -> Bus Creator3/7  "Tire_Out SideFrc"
  TireFL/6(LongFrc) -> Bus Creator3/6  "Tire_Out LongFrc"
  TireFL/5(vBelt) -> Bus Creator3/5  "Tire_Out vBelt"
  TireFL/4(rBelt_eff) -> Bus Creator3/4  "Tire_Out rBelt_eff"
  TireFL/3(TurnSlp) -> Bus Creator3/3  "Tire_Out TurnSlp"
  TireFL/1(Slp) -> Bus Creator3/1  "Tire_Out Slp"
  TireFL/2(Alpha) -> Bus Creator3/2  "Tire_Out Alpha"
  Bus Creator3/1 -> TireFL_Out/1
  TireFR_In/1 -> Demux1/1
  TireRL_In/1 -> Demux2/1
  TireRR_In/1 -> Demux3/1

== system generic/CarMaker/IPG Vehicle/CarAndTrailer/Forces/Vehicle Forces ==
  Sync_In : Inport
  Bus Creator1 : BusCreator  Inputs=12
  Bus Creator8 : BusCreator  Inputs=16
  BusCreator1 : BusCreator  Inputs=4
  BusCreator2 : BusCreator  Inputs=9
  Demux : Demux  Outputs=16
      settings: DisplayOption=none
  Demux1 : Demux  Outputs=12
      settings: DisplayOption=none
  Demux2 : Demux  Outputs=13
      settings: DisplayOption=none
  Forces : S-Function  FunctionName=CM_Sfun  Parameters='Forces'  SFunctionDeploymentMode=off  EnableBusSupport=off
  Terminator : Terminator
  Sync_Out : Outport  VectorParamsAs1DForOutWhenUnconnected=off
  Car.Virtual : Outport  Port=2  VectorParamsAs1DForOutWhenUnconnected=off
  Car.Aero : Outport  Port=3  VectorParamsAs1DForOutWhenUnconnected=off
  Car.Load : Outport  Port=4  VectorParamsAs1DForOutWhenUnconnected=off
  wires:
  BusCreator1/1 -> Terminator/1  "Aero IF (in)"
  Demux2/13 -> BusCreator2/9  "car Aero Trq_1 z"
  Demux2/12 -> BusCreator2/8  "car Aero Trq_1 y"
  Demux2/11 -> BusCreator2/7  "car Aero Trq_1 x"
  Demux2/10 -> BusCreator2/6  "car Aero Frc_1 z"
  Demux2/9 -> BusCreator2/5  "car Aero Frc_1 y"
  Demux2/8 -> BusCreator2/4  "car Aero Frc_1 x"
  Demux2/7 -> BusCreator2/3  "car Aero PoA_1 z"
  Demux2/6 -> BusCreator2/2  "car Aero PoA_1 y"
  Demux2/5 -> BusCreator2/1  "car Aero PoA_1 x"
  Demux2/4 -> BusCreator1/4  "car Aero tau_1"
  Demux2/3 -> BusCreator1/3  "car Aero ApproachVel_1 z"
  Demux2/2 -> BusCreator1/2  "car Aero ApproachVel_1 y"
  Demux2/1 -> BusCreator1/1  "car Aero ApproachVel_1 x"
  Demux/16 -> Bus Creator8/16  "Car Load_3 tz"
  Demux/15 -> Bus Creator8/15  "Car Load_3 ty"
  Demux/14 -> Bus Creator8/14  "Car Load_3 tx"
  Demux/13 -> Bus Creator8/13  "Car Load_3 mass"
  Demux1/12 -> Bus Creator1/12  "Car Virtual Trq_0 z"
  Demux1/11 -> Bus Creator1/11  "Car Virtual Trq_0 y"
  Demux1/10 -> Bus Creator1/10  "Car Virtual Trq_0 x"
  Demux1/9 -> Bus Creator1/9  "Car Virtual Trq_1 z"
  Demux1/8 -> Bus Creator1/8  "Car Virtual Trq_1 y"
  Demux1/7 -> Bus Creator1/7  "Car Virtual Trq_1 x"
  Demux1/6 -> Bus Creator1/6  "Car Virtual Frc_0 z"
  Demux1/5 -> Bus Creator1/5  "Car Virtual Frc_0 y"
  Demux1/4 -> Bus Creator1/4  "Car Virtual Frc_0 x"
  Sync_In/1 -> Forces/1
  Forces/1 -> Sync_Out/1
  BusCreator2/1 -> Car.Aero/1
  Demux1/1 -> Bus Creator1/1  "Car Virtual Frc_1 x"
  Demux1/2 -> Bus Creator1/2  "Car Virtual Frc_1 y"
  Demux1/3 -> Bus Creator1/3  "Car Virtual Frc_1 z"
  Forces/3 -> Demux2/1
  Forces/2 -> Demux1/1
  Bus Creator1/1 -> Car.Virtual/1
  Bus Creator8/1 -> Car.Load/1
  Demux/1 -> Bus Creator8/1  "Car Load_0 mass"
  Demux/2 -> Bus Creator8/2  "Car Load_0 tx"
  Demux/3 -> Bus Creator8/3  "Car Load_0 ty"
  Demux/4 -> Bus Creator8/4  "Car Load_0 tz"
  Demux/5 -> Bus Creator8/5  "Car Load_1 mass"
  Demux/6 -> Bus Creator8/6  "Car Load_1 tx"
  Demux/7 -> Bus Creator8/7  "Car Load_1 ty"
  Demux/8 -> Bus Creator8/8  "Car Load_1 tz"
  Demux/9 -> Bus Creator8/9  "Car Load_2 mass"
  Demux/10 -> Bus Creator8/10  "Car Load_2 tx"
  Demux/11 -> Bus Creator8/11  "Car Load_2 ty"
  Demux/12 -> Bus Creator8/12  "Car Load_2 tz"
  Forces/4 -> Demux/1

== system generic/CarMaker/IPG Vehicle/CarAndTrailer/Trailer/CreateBus Car.Hitch.FrcTrq ==
  In1 : Inport
  Bus Creator7 : BusCreator  Inputs=6
  Demux7 : Demux  Outputs=6
      settings: DisplayOption=none
  Out1 : Outport  VectorParamsAs1DForOutWhenUnconnected=off
  wires:
  In1/1 -> Demux7/1
  Bus Creator7/1 -> Out1/1
  Demux7/6 -> Bus Creator7/6  "Car Hitch Trq2Car z"
  Demux7/5 -> Bus Creator7/5  "Car Hitch Trq2Car y"
  Demux7/4 -> Bus Creator7/4  "Car Hitch Trq2Car x"
  Demux7/3 -> Bus Creator7/3  "Car Hitch Frc2Car z"
  Demux7/2 -> Bus Creator7/2  "Car Hitch Frc2Car y"
  Demux7/1 -> Bus Creator7/1  "Car Hitch Frc2Car x"

== system generic/CarMaker/IPG Vehicle/CarAndTrailer/Trailer/CreateBus Vhcl.Motion ==
  In1 : Inport
  BusCreator : BusCreator  Inputs=15
  Demux : Demux  Outputs=15
      settings: DisplayOption=none
  Out1 : Outport  VectorParamsAs1DForOutWhenUnconnected=off
  wires:
  Demux/15 -> BusCreator/15  "Vhcl YawAcc"
  Demux/14 -> BusCreator/14  "Vhcl YawVel"
  Demux/13 -> BusCreator/13  "Vhcl Yaw"
  Demux/12 -> BusCreator/12  "Vhcl PitchAcc"
  Demux/11 -> BusCreator/11  "Vhcl PitchVel"
  Demux/10 -> BusCreator/10  "Vhcl Pitch"
  Demux/9 -> BusCreator/9  "Vhcl RollAcc"
  Demux/8 -> BusCreator/8  "Vhcl RollVel"
  Demux/7 -> BusCreator/7  "Vhcl Roll"
  Demux/6 -> BusCreator/6  "Vhcl Hitch_Pos z"
  Demux/5 -> BusCreator/5  "Vhcl Hitch_Pos y"
  Demux/4 -> BusCreator/4  "Vhcl Hitch_Pos x"
  Demux/3 -> BusCreator/3  "Vhcl sRoad"
  Demux/2 -> BusCreator/2  "Vhcl Distance"
  Demux/1 -> BusCreator/1  "Vhcl v"
  In1/1 -> Demux/1
  BusCreator/1 -> Out1/1

== system generic/CarMaker/IPG Vehicle/CarAndTrailer/Trailer/CreateBus Vhcl.PoI ==
  In1 : Inport
  Bus Creator3 : BusCreator  Inputs=18
  Demux3 : Demux  Outputs=18
      settings: DisplayOption=none
  Out1 : Outport  VectorParamsAs1DForOutWhenUnconnected=off
  wires:
  Demux3/18 -> Bus Creator3/18  "Vhcl PoI_GCS Elev"
  Demux3/17 -> Bus Creator3/17  "Vhcl PoI_GCS Lat"
  Demux3/16 -> Bus Creator3/16  "Vhcl PoI_GCS Long"
  Demux3/15 -> Bus Creator3/15  "Vhcl PoI_Acc_1 z"
  Demux3/14 -> Bus Creator3/14  "Vhcl PoI_Acc_1 y"
  Demux3/13 -> Bus Creator3/13  "Vhcl PoI_Acc_1 x"
  Demux3/12 -> Bus Creator3/12  "Vhcl PoI_Vel_1 z"
  Demux3/11 -> Bus Creator3/11  "Vhcl PoI_Vel_1 y"
  Demux3/10 -> Bus Creator3/10  "Vhcl PoI_Vel_1 x"
  Demux3/9 -> Bus Creator3/9  "Vhcl PoI_Acc z"
  Demux3/8 -> Bus Creator3/8  "Vhcl PoI_Acc y"
  Demux3/7 -> Bus Creator3/7  "Vhcl PoI_Acc x"
  Demux3/6 -> Bus Creator3/6  "Vhcl PoI_Vel z"
  Demux3/5 -> Bus Creator3/5  "Vhcl PoI_Vel y"
  Demux3/4 -> Bus Creator3/4  "Vhcl PoI_Vel x"
  Demux3/3 -> Bus Creator3/3  "Vhcl PoI_Pos z"
  Demux3/2 -> Bus Creator3/2  "Vhcl PoI_Pos y"
  In1/1 -> Demux3/1
  Bus Creator3/1 -> Out1/1
  Demux3/1 -> Bus Creator3/1  "Vhcl PoI_Pos x"

== system generic/CarMaker/IPG Vehicle/CarAndTrailer/Trailer/CreateBus Vhcl.Steering ==
  In1 : Inport
  Bus Creator3 : BusCreator  Inputs=4
  Demux : Demux
      settings: DisplayOption=none
  Out1 : Outport  VectorParamsAs1DForOutWhenUnconnected=off
  wires:
  Bus Creator3/1 -> Out1/1
  Demux/1 -> Bus Creator3/1  "Vhcl Steering Ang"
  Demux/3 -> Bus Creator3/3  "Vhcl Steering AngAcc"
  Demux/2 -> Bus Creator3/2  "Vhcl Steering AngVel"
  Demux/4 -> Bus Creator3/4  "Vhcl Steering Trq"
  In1/1 -> Demux/1

== system generic/CarMaker/IPG Vehicle/CarAndTrailer/Trailer/CreateBus Vhcl.Wheel.FL ==
  In1 : Inport
  Bus Creator3 : BusCreator  Inputs=14
  Demux3 : Demux  Outputs=14
      settings: DisplayOption=none
  Out1 : Outport  VectorParamsAs1DForOutWhenUnconnected=off
  wires:
  Demux3/14 -> Bus Creator3/14  "Vhcl Wheel FL Trq_WhlBearing"
  Demux3/13 -> Bus Creator3/13  "Vhcl Wheel FL Trq_T2W"
  Demux3/12 -> Bus Creator3/12  "Vhcl Wheel FL SideSlip"
  Demux3/11 -> Bus Creator3/11  "Vhcl Wheel FL LongSlip"
  Demux3/10 -> Bus Creator3/10  "Vhcl Wheel FL vBelt"
  Demux3/9 -> Bus Creator3/9  "Vhcl Wheel FL Fz"
  Demux3/8 -> Bus Creator3/8  "Vhcl Wheel FL Fy"
  Demux3/7 -> Bus Creator3/7  "Vhcl Wheel FL Fx"
  Demux3/6 -> Bus Creator3/6  "Vhcl Wheel FL r_zxy z"
  Demux3/5 -> Bus Creator3/5  "Vhcl Wheel FL r_zxy y"
  Demux3/4 -> Bus Creator3/4  "Vhcl Wheel FL r_zxy x"
  Demux3/3 -> Bus Creator3/3  "Vhcl Wheel FL t z"
  Demux3/2 -> Bus Creator3/2  "Vhcl Wheel FL t y"
  In1/1 -> Demux3/1
  Bus Creator3/1 -> Out1/1
  Demux3/1 -> Bus Creator3/1  "Vhcl Wheel FL t x"

== system generic/CarMaker/IPG Vehicle/CarAndTrailer/Trailer/CreateBus Vhcl.Wheel.FR ==
  In1 : Inport
  Bus Creator3 : BusCreator  Inputs=14
  Demux3 : Demux  Outputs=14
      settings: DisplayOption=none
  Out1 : Outport  VectorParamsAs1DForOutWhenUnconnected=off
  wires:
  Demux3/14 -> Bus Creator3/14  "Vhcl Wheel FR Trq_WhlBearing"
  Demux3/13 -> Bus Creator3/13  "Vhcl Wheel FR Trq_T2W"
  Demux3/12 -> Bus Creator3/12  "Vhcl Wheel FR SideSlip"
  Demux3/11 -> Bus Creator3/11  "Vhcl Wheel FR LongSlip"
  Demux3/10 -> Bus Creator3/10  "Vhcl Wheel FR vBelt"
  Demux3/9 -> Bus Creator3/9  "Vhcl Wheel FR Fz"
  Demux3/8 -> Bus Creator3/8  "Vhcl Wheel FR Fy"
  Demux3/7 -> Bus Creator3/7  "Vhcl Wheel FR Fx"
  Demux3/6 -> Bus Creator3/6  "Vhcl Wheel FR r_zxy z"
  Demux3/5 -> Bus Creator3/5  "Vhcl Wheel FR r_zxy y"
  Demux3/4 -> Bus Creator3/4  "Vhcl Wheel FR r_zxy x"
  Demux3/3 -> Bus Creator3/3  "Vhcl Wheel FR t z"
  Demux3/2 -> Bus Creator3/2  "Vhcl Wheel FR t y"
  In1/1 -> Demux3/1
  Bus Creator3/1 -> Out1/1
  Demux3/1 -> Bus Creator3/1  "Vhcl Wheel FR t x"

== system generic/CarMaker/IPG Vehicle/CarAndTrailer/Trailer/CreateBus Vhcl.Wheel.RL ==
  In1 : Inport
  Bus Creator3 : BusCreator  Inputs=14
  Demux3 : Demux  Outputs=14
      settings: DisplayOption=none
  Out1 : Outport  VectorParamsAs1DForOutWhenUnconnected=off
  wires:
  Demux3/14 -> Bus Creator3/14  "Vhcl Wheel RL Trq_WhlBearing"
  Demux3/13 -> Bus Creator3/13  "Vhcl Wheel RL Trq_T2W"
  Demux3/12 -> Bus Creator3/12  "Vhcl Wheel RL SideSlip"
  Demux3/11 -> Bus Creator3/11  "Vhcl Wheel RL LongSlip"
  Demux3/10 -> Bus Creator3/10  "Vhcl Wheel RL vBelt"
  Demux3/9 -> Bus Creator3/9  "Vhcl Wheel RL Fz"
  Demux3/8 -> Bus Creator3/8  "Vhcl Wheel RL Fy"
  Demux3/7 -> Bus Creator3/7  "Vhcl Wheel RL Fx"
  Demux3/6 -> Bus Creator3/6  "Vhcl Wheel RL r_zxy z"
  Demux3/5 -> Bus Creator3/5  "Vhcl Wheel RL r_zxy y"
  Demux3/4 -> Bus Creator3/4  "Vhcl Wheel RL r_zxy x"
  Demux3/3 -> Bus Creator3/3  "Vhcl Wheel RL t z"
  Demux3/2 -> Bus Creator3/2  "Vhcl Wheel RL t y"
  In1/1 -> Demux3/1
  Bus Creator3/1 -> Out1/1
  Demux3/1 -> Bus Creator3/1  "Vhcl Wheel RL t x"

== system generic/CarMaker/IPG Vehicle/CarAndTrailer/Trailer/CreateBus Vhcl.Wheel.RR ==
  In1 : Inport
  Bus Creator3 : BusCreator  Inputs=14
  Demux3 : Demux  Outputs=14
      settings: DisplayOption=none
  Out1 : Outport  VectorParamsAs1DForOutWhenUnconnected=off
  wires:
  Demux3/14 -> Bus Creator3/14  "Vhcl Wheel RR Trq_WhlBearing"
  Demux3/13 -> Bus Creator3/13  "Vhcl Wheel RR Trq_T2W"
  Demux3/12 -> Bus Creator3/12  "Vhcl Wheel RR SideSlip"
  Demux3/11 -> Bus Creator3/11  "Vhcl Wheel RR LongSlip"
  Demux3/10 -> Bus Creator3/10  "Vhcl Wheel RR vBelt"
  Demux3/9 -> Bus Creator3/9  "Vhcl Wheel RR Fz"
  Demux3/8 -> Bus Creator3/8  "Vhcl Wheel RR Fy"
  Demux3/7 -> Bus Creator3/7  "Vhcl Wheel RR Fx"
  Demux3/6 -> Bus Creator3/6  "Vhcl Wheel RR r_zxy z"
  Demux3/5 -> Bus Creator3/5  "Vhcl Wheel RR r_zxy y"
  Demux3/4 -> Bus Creator3/4  "Vhcl Wheel RR r_zxy x"
  Demux3/3 -> Bus Creator3/3  "Vhcl Wheel RR t z"
  Demux3/2 -> Bus Creator3/2  "Vhcl Wheel RR t y"
  In1/1 -> Demux3/1
  Bus Creator3/1 -> Out1/1
  Demux3/1 -> Bus Creator3/1  "Vhcl Wheel RR t x"

== system generic/CarMaker/VehicleControl/CreateBus VhclCtrl1/A*algoithm/Subsystem ==
  Bus Selector : BusSelector  OutputSignals=Route.tx,Route.ty
  Constant : Constant  Value=0
  Constant1 : Constant  Value=0
  Read CM Dict : CarMaker4SL/Read CM Dict  xname=Sensor.Radar.VehSensor_6.Obj0.DistX  xsync=off  xstime=Continuous
  Read CM Dict1 : CarMaker4SL/Read CM Dict  xname=Sensor.Radar.VehSensor_6.Obj0.DistY  xsync=off  xstime=Continuous
  Read CM Dict3 : CarMaker4SL/Read CM Dict  xname=Sensor.Radar.VehSensor_6.Obj0.ProbObst  xsync=off  xstime=Continuous
  Road Sensor : CarMaker4SL/Sensors/Road Sensor  xname=0  xstime=Continuous
      settings: SourceProductName=CarMaker4SL
  Sum : Sum  Inputs=|++
  Sum1 : Sum  Inputs=|++
  Switch : Switch  Criteria=u2 > Threshold  SaturateOnIntegerOverflow=off  InputSameDT=off
  Switch1 : Switch  Criteria=u2 > Threshold  SaturateOnIntegerOverflow=off  InputSameDT=off
  Out1 : Outport
  Out2 : Outport  Port=2
  Out3 : Outport  Port=3
  wires:
  Read CM Dict1/1 -> Sum/1
  Sum/1 -> Switch/1
  Constant/1 -> Switch1/3, Switch/3
  Sum1/1 -> Switch1/1
  Switch/1 -> Out1/1
  Bus Selector/2 -> Sum1/1  "<ty>"
  Read CM Dict3/1 -> Switch1/2, Switch/2
  Read CM Dict/1 -> Sum1/2
  Road Sensor/2 -> Bus Selector/1
  Constant1/1 -> Road Sensor/1
  Bus Selector/1 -> Sum/2  "<tx>"
  Road Sensor/1 -> Out3/1
  Switch1/1 -> Out2/1

== system generic/CarMaker/VehicleControl/CreateBus VhclCtrl1/MPC_steering_controllers/State_space_system_variables ==
  Yaw_ref_deg : Inport
  <ty> : Inport  Port=2
  Discrete-Time Integrator2 : DiscreteIntegrator  SampleTime=-1  ICPrevOutput=DiscIntNeverNeededParam  ICPrevScaledInput=DiscIntNeverNeededParam
  Gain : Gain  Gain=3.6
  Mux : Mux  Inputs=8
  Radians to Degrees2 : simulink_extras/Transformations/Radians to Degrees
  Radians to Degrees3 : simulink_extras/Transformations/Radians to Degrees
  Read CM Dict10 : CarMaker4SL/Read CM Dict  xname=Car.Gen.tx  xsync=off  xstime=Continuous
  Read CM Dict2 : CarMaker4SL/Read CM Dict  xname=Car.YawRate  xsync=off  xstime=Continuous
  Read CM Dict3 : CarMaker4SL/Read CM Dict  xname=Car.YawRate  xsync=off  xstime=Continuous
  Read CM Dict4 : CarMaker4SL/Read CM Dict  xname=Car.Gen.tx  xsync=off  xstime=Continuous
  Read CM Dict5 : CarMaker4SL/Read CM Dict  xname=Car.Gen.ty  xsync=off  xstime=Continuous
  Read CM Dict6 : CarMaker4SL/Read CM Dict  xname=Car.Con.vy_1  xsync=off  xstime=Continuous
  Read CM Dict7 : CarMaker4SL/Read CM Dict  xname=Car.Con.vx_1  xsync=off  xstime=Continuous
  Sum : Sum  Inputs=|++
  Terminator : Terminator
  Vlocity_correction : Constant
  x : Outport
  Lateral_velocity : Outport  Port=2
  wires:
  Vlocity_correction/1 -> Sum/2
  Read CM Dict4/1 -> Terminator/1
  Read CM Dict2/1 -> Discrete-Time Integrator2/1
  Radians to Degrees3/1 -> Mux/2
  Discrete-Time Integrator2/1 -> Radians to Degrees3/1
  Read CM Dict6/1 -> Gain/1
  Read CM Dict3/1 -> Radians to Degrees2/1
  Read CM Dict7/1 -> Sum/1  "Longitudinal_velocity"
  Gain/1 -> Mux/1, Lateral_velocity/1
  Radians to Degrees2/1 -> Mux/3
  Read CM Dict5/1 -> Mux/4
  Read CM Dict10/1 -> Mux/5
  <ty>/1 -> Mux/6
  Yaw_ref_deg/1 -> Mux/7
  Sum/1 -> Mux/8
  Mux/1 -> x/1  "x"

== system generic/CarMaker/VehicleControl/CreateBus VhclCtrl1/MPC_steering_controllers/Subsystem ==
  x : Inport
  u : Inport  Port=2
  dt : Inport  Port=3
  dev : Inport  Port=4
  Constant4 : Constant  Commented=on  Value=B
  Constant5 : Constant  Value=21543*180/pi()
  Constant6 : Constant  Value=70551*180/pi()
  MATLAB Function1 : MATLAB Function  Commented=on  TreatAsAtomicUnit=on
  MATLAB Function2 : MATLAB Function  Commented=on  TreatAsAtomicUnit=on
  MATLAB Function3 : MATLAB Function  Commented=on  TreatAsAtomicUnit=on
  MATLAB Function4 : MATLAB Function  Commented=on  TreatAsAtomicUnit=on
  MATLAB Function5 : MATLAB Function  Commented=on  TreatAsAtomicUnit=on
  MATLAB Function6 : MATLAB Function  Commented=on  TreatAsAtomicUnit=on
  MATLAB Function7 : MATLAB Function  Commented=on  TreatAsAtomicUnit=on
  S-Function : S-Function  Commented=on  FunctionName=MPCController2  SFunctionDeploymentMode=off  EnableBusSupport=off
  u_optimal : Outport
  steering : Outport  Port=2
  x_new : Outport  Port=3
  theta_new : Outport  Port=4
  wires:
  Constant4/1 -> MATLAB Function1/2(B)
  dt/1 -> MATLAB Function3/3(dt)
  u/1 -> MATLAB Function3/2(u)
  x/1 -> MATLAB Function3/1(x)
  MATLAB Function3/1(u_optimal) -> u_optimal/1
  MATLAB Function3/3(theta_new) -> theta_new/1
  MATLAB Function1/1(steering) -> steering/1
  MATLAB Function3/2(x_new) -> x_new/1
  dev/1 -> MATLAB Function1/1(dev)
  MATLAB Function2/1(delta) -> ?

== system generic/CarMaker/VehicleControl/CreateBus VhclCtrl1/MPC_steering_controllers/Tradition_MPC ==
  Lateral_deviation : Inport
  Dev_angle : Inport  Port=2
  Constant8 : Constant  Value=A
  Constant9 : Constant  Value=B
  MPC_steering_control : MATLAB Function  TreatAsAtomicUnit=on
  MPC_steering_control1 : MATLAB Function  TreatAsAtomicUnit=on
  Sum1 : Sum  Inputs=|++
  steering_cmd : Outport
  wires:
  MPC_steering_control/1(steering_cmd) -> Sum1/1
  Sum1/1 -> steering_cmd/1
  Constant8/1 -> MPC_steering_control1/2(A), MPC_steering_control/2(A)
  MPC_steering_control1/1(steering_cmd) -> Sum1/2
  Constant9/1 -> MPC_steering_control1/3(B), MPC_steering_control/3(B)
  Dev_angle/1 -> MPC_steering_control1/1(Heading_error)
  Lateral_deviation/1 -> MPC_steering_control/1(Lateral_deviation)

== system generic/CarMaker/VehicleControl/CreateBus VhclCtrl1/PID steering controller/Dervative ==
  Error : Inport
  Discrete Derivative : simulink/Discrete/Discrete Derivative  gainval=1.0  ICPrevScaledInput=0.01  OutMin=[]  OutMax=[]  OutDataType=fixdt(1, 16)  OutScaling=2^-10  DoSatur=off
  Gain2 : Gain  Gain=0.4
  Dervative term : Outport
  wires:
  Error/1 -> Gain2/1
  Gain2/1 -> Discrete Derivative/1
  Discrete Derivative/1 -> Dervative term/1

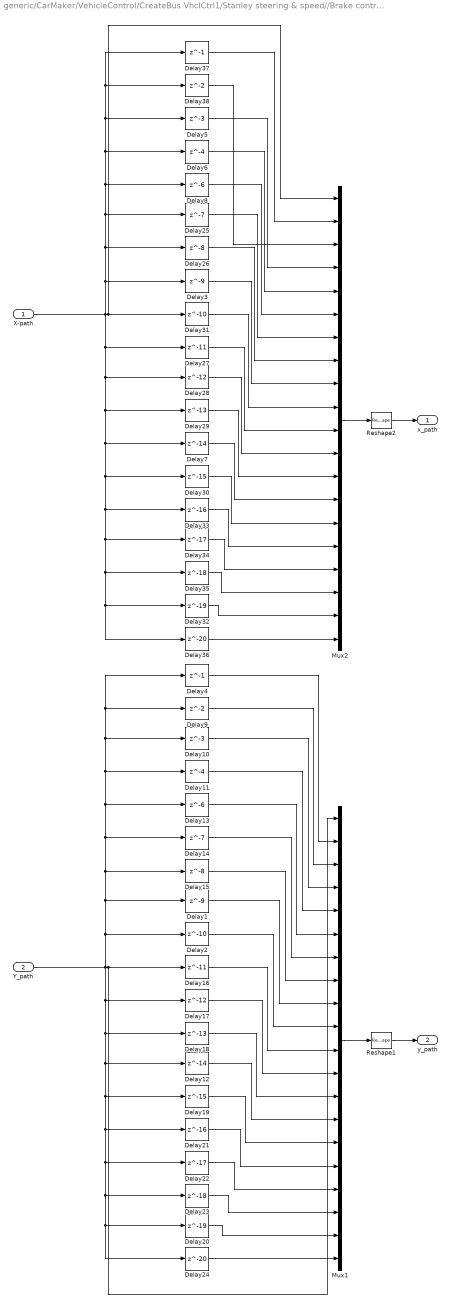
== system generic/CarMaker/VehicleControl/CreateBus VhclCtrl1/Stanley steering & speed//Brake controller/ Path_expanding ==
  X-path : Inport
  Y_path : Inport  Port=2
  Delay1 : Delay  DelayLength=9
  Delay10 : Delay  DelayLength=3
  Delay11 : Delay  DelayLength=4
  Delay12 : Delay  DelayLength=14
  Delay13 : Delay  DelayLength=6
  Delay14 : Delay  DelayLength=7
  Delay15 : Delay  DelayLength=8
  Delay16 : Delay  DelayLength=11
  Delay17 : Delay  DelayLength=12
  Delay18 : Delay  DelayLength=13
  Delay19 : Delay  DelayLength=15
  Delay2 : Delay  DelayLength=10
  Delay20 : Delay  DelayLength=19
  Delay21 : Delay  DelayLength=16
  Delay22 : Delay  DelayLength=17
  Delay23 : Delay  DelayLength=18
  Delay24 : Delay  DelayLength=20
  Delay25 : Delay  DelayLength=7
  Delay26 : Delay  DelayLength=8
  Delay27 : Delay  DelayLength=11
  Delay28 : Delay  DelayLength=12
  Delay29 : Delay  DelayLength=13
  Delay3 : Delay  DelayLength=9
  Delay30 : Delay  DelayLength=15
  Delay31 : Delay  DelayLength=10
  Delay32 : Delay  DelayLength=19
  Delay33 : Delay  DelayLength=16
  Delay34 : Delay  DelayLength=17
  Delay35 : Delay  DelayLength=18
  Delay36 : Delay  DelayLength=20
  Delay37 : Delay  DelayLength=1
  Delay38 : Delay
  Delay4 : Delay  DelayLength=1
  Delay5 : Delay  DelayLength=3
  Delay6 : Delay  DelayLength=4
  Delay7 : Delay  DelayLength=14
  Delay8 : Delay  DelayLength=6
  Delay9 : Delay
  Mux1 : Mux  Inputs=20
  Mux2 : Mux  Inputs=20
  Reshape1 : Reshape  OutputDimensionality=Customize  OutputDimensions=[1,20]
  Reshape2 : Reshape  OutputDimensionality=Customize  OutputDimensions=[1,20]
  x_path : Outport
  y_path : Outport  Port=2
  wires:
  Delay12/1 -> Mux1/14
  X-path/1 -> Delay32/1, Delay36/1, Delay35/1, Delay34/1, Delay33/1, Delay30/1, Delay7/1, Delay29/1, Delay28/1, Delay27/1, Delay31/1, Mux2/1, Delay38/1, Delay37/1, Delay5/1, Delay6/1, Delay8/1, Delay25/1, Delay26/1, Delay3/1
  Delay25/1 -> Mux2/7
  Delay17/1 -> Mux1/12
  Y_path/1 -> Delay20/1, Delay24/1, Delay23/1, Delay22/1, Delay21/1, Delay19/1, Delay12/1, Delay18/1, Delay17/1, Mux1/1, Delay16/1, Delay4/1, Delay9/1, Delay10/1, Delay11/1, Delay13/1, Delay14/1, Delay15/1, Delay1/1, Delay2/1
  Delay5/1 -> Mux2/4
  Delay37/1 -> Mux2/2
  Delay6/1 -> Mux2/5
  Delay38/1 -> Mux2/3
  Delay20/1 -> Mux1/19
  Delay18/1 -> Mux1/13
  Delay8/1 -> Mux2/6
  Delay26/1 -> Mux2/8
  Delay3/1 -> Mux2/9
  Delay31/1 -> Mux2/10
  Delay27/1 -> Mux2/11
  Delay24/1 -> Mux1/20
  Delay28/1 -> Mux2/12
  Delay29/1 -> Mux2/13
  Delay7/1 -> Mux2/14
  Delay30/1 -> Mux2/15
  Delay33/1 -> Mux2/16
  Mux1/1 -> Reshape1/1
  Delay34/1 -> Mux2/17
  Delay35/1 -> Mux2/18
  Delay1/1 -> Mux1/9
  Delay32/1 -> Mux2/19
  Delay15/1 -> Mux1/8
  Delay36/1 -> Mux2/20
  Reshape1/1 -> y_path/1
  Delay4/1 -> Mux1/2
  Delay16/1 -> Mux1/11
  Delay9/1 -> Mux1/3
  Delay21/1 -> Mux1/16
  Delay10/1 -> Mux1/4
  Delay11/1 -> Mux1/5
  Delay13/1 -> Mux1/6
  Reshape2/1 -> x_path/1
  Delay14/1 -> Mux1/7
  Delay2/1 -> Mux1/10
  Delay19/1 -> Mux1/15
  Delay22/1 -> Mux1/17
  Delay23/1 -> Mux1/18
  Mux2/1 -> Reshape2/1

== system generic/CarMaker/VehicleControl/CreateBus VhclCtrl1/Stanley steering & speed//Brake controller/Road sensor set & path planning ==
  Road sensor set & path planning : Subsystem  VariantControl=Choice
  <tx> : Outport
  <ty> : Outport  Port=2
  <DevDist> : Outport  Port=3
  <CurveXY> : Outport  Port=4
  Yaw_rate : Outport  Port=5
  Velocity_m_s : Outport  Port=6
  smoothed_path_curvature : Outport  Port=7

== system generic/CarMaker/VehicleControl/CreateBus VhclCtrl1/Stanley steering & speed//Brake controller/Stanley controller version_1 ==
  Direction : Inport
  Stanley controller version_1 : Subsystem  VariantControl=Choice  ReferencedSubsystem=Stanley_controller_version_1
  Radians out : Outport
  SteerCmd : Outport  Port=2

== system generic/CarMaker/VehicleControl/CreateBus VhclCtrl1/Stanley steering & speed//Brake controller/Stanley controller with path_planning ==
  X-path : Inport
  Y_path : Inport  Port=2
  Stanley controller with path_planning : Subsystem  VariantControl=Choice
  e : Outport
  err_fr_axle : Outport  Port=2
  cross_track_steering : Outport  Port=3
  heading_err : Outport  Port=4
  Steering : Outport  Port=5
  closest_point : Outport  Port=6

== system generic/CarMaker/VehicleControl/CreateBus VhclCtrl1/Stanley steering & speed//Brake controller/Stanley_controller_vfin ==
  Velocity : Inport
  Curvature : Inport  Port=2
  Vehicle_yaw_rate : Inport  Port=3
  Path.DevDist : Inport  Port=4
  Stanley_controller_vfin : Subsystem  Variant=on  VariantControlMode=label  VariantControl=Choice  LabelModeActiveChoice=Choice
  Steering angle : Outport
  dev_angle : Outport  Port=2
